simulink model "NDM200"  (Simulink 7.6)
settings: Solver=ode45  StartTime=0.0  StopTime=SimulTime  RelTol=1e-3
values from neighbouring files (symbols this model uses):
  T_amb = 296    [Parameters.m]
undefined symbols (not defined in the file or in its folder): Job
libraries: simulink x1, WZM_QSS_Lib x1
settings Model: Creator=simon  LastModifiedBy=conid
settings DebuggingCC: AlgebraicLoopMsg=none  SolverPrmCheckMsg=none

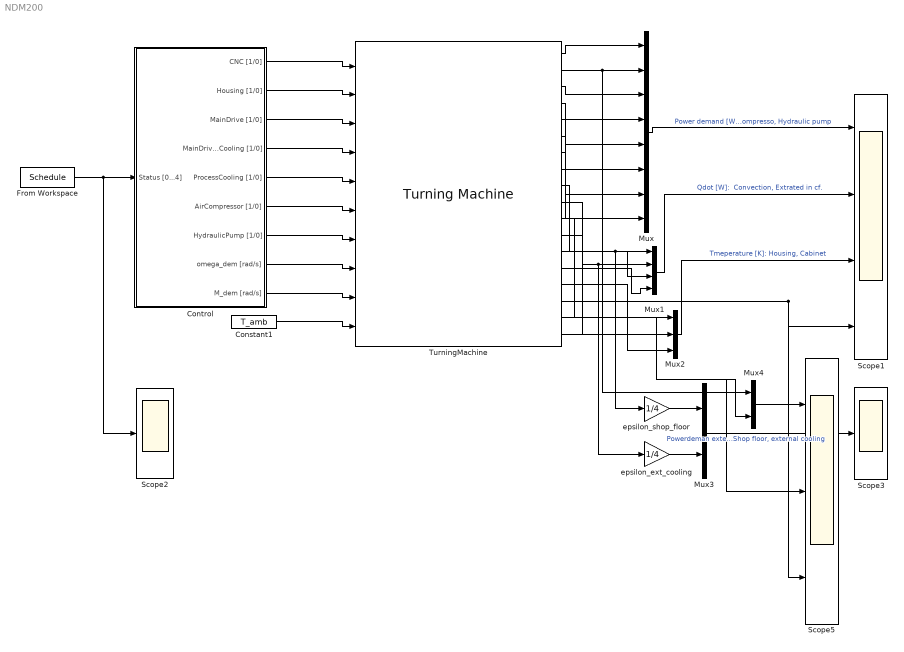
== system NDM200 ==
  Constant1 : Constant  Value=T_amb
  Control : Subsystem  mask{CNC=[0 1 1 1 1], Housing=[0 1 1 1 1], MainDrive=[0 0 0 0 1], MainDriveCooling=[0 0 1 1 1], ProcessCooling=[0 0 0 0 1], AirCompressor=[0 0 1 1 1], HydraulicPump=[0 0 1 1 1], Job=Job}
      mask prompts: CNC "Cabinet"; MainDrive "Main drive"; MainDriveCooling "Main drive cooling"; ProcessCooling "Process cooling"; Job "Job struct"
      mask help:
      | Controls the components of the machine:
      |
      | Status:
      |     0. Off
      |     1. Standby
      |     2. Warmup
      |     3. Setting
      |     4. Machining
      |
      | If the status is machining, the job defined as
      |     - Job.time
      |     - Job.omega_dem
      |     - Job.M_dem
      | will be runned, and repeated.
      mask TabNameString: Status,Status,Status,Status,Status,Status,Status,Job
  From Workspace : FromWorkspace  VariableName=Schedule  SampleTime=0  Interpolate=off  OutputAfterFinalValue=Holding final value
  Mux : Mux  Inputs=8
  Mux1 : Mux
  Mux2 : Mux  Inputs=3
  Mux3 : Mux  Inputs=2
  Mux4 : Mux  Inputs=2
  Scope1 : Scope  NumInputPorts=4
      settings: TickLabels=on  TimeRange=1000  YMin=0~-3e+008~215~-3.25e+010  YMax=200000~1.1e+009~295~2.5e+009  SaveName=Scp_Main
  Scope2 : Scope
      settings: TickLabels=on  TimeRange=350  YMin=0.95  YMax=1.05  SaveName=Scp_Schedule
  Scope3 : Scope
      settings: TickLabels=on  TimeRange=350  YMin=-2.5e+13  YMax=1.25e+13  SaveName=Scp_PwrExt
  Scope5 : Scope  NumInputPorts=3
      settings: TickLabels=on  TimeRange=2000  YMin=0~0~296  YMax=12486.03351955308~5000~306  SaveName=Scp_Main1
  TurningMachine : WZM_QSS_Lib/Assembly/Turning Machine  SystemSampleTime=-1  MainDrive=MainDrive  MainDriveCoolingEx=MainDriveCoolingEx  CNC=CNC  Process=Process  ProcessCooling=ProcessCooling  Housing=Housing  AirCompressor=AirCompressor  HydraulicPump=HydraulicPump  LocMainDrive=machine housing  LocProcessCooling=shop floor  LocProcess=process housing  LocMachine=shop floor  LocMachineExtr=shop floor  LocCNC=shop floor  LocCNCExtr=shop floor  LocAirCompressor=shop floor  LocHydraulicPump=shop floor
      link override MainDrive/MainDrive_simple/Lookup Table (n-D): InterpMethod=Cubic spline
  epsilon_ext_cooling : Gain  Gain=1/4
  epsilon_shop_floor : Gain  Gain=1/4
  wires:
  TurningMachine/1 -> Mux/1
  TurningMachine/2 -> Mux/2, Mux4/1
  TurningMachine/3 -> Mux/3
  TurningMachine/4 -> Mux/4
  TurningMachine/5 -> Mux/5
  TurningMachine/6 -> Mux/6
  Mux/1 -> Scope1/1  "Power demand [W]: Total,  CNC, Main Drive Cooling,  Housing, Process cooling, Cabinet cooling, Air compresso, Hydraulic pump"
  Mux1/1 -> Scope1/2  "Qdot [W]:  Convection, Extrated in cf."
  Mux2/1 -> Scope1/3  "Tmeperature [K]: Housing, Cabinet"
  TurningMachine/7 -> Mux/7
  TurningMachine/8 -> Mux/8
  TurningMachine/9 -> Mux1/1, epsilon_shop_floor/1
  TurningMachine/10 -> epsilon_ext_cooling/1, Mux1/2
  TurningMachine/11 -> Mux2/1
  TurningMachine/12 -> Mux2/2
  Control/1(CNC [1/0]) -> TurningMachine/1
  Control/2(Housing [1/0]) -> TurningMachine/2
  Control/3(MainDrive [1/0]) -> TurningMachine/3
  Control/4(MainDriveCooling [1/0]) -> TurningMachine/4
  Control/5(ProcessCooling [1/0]) -> TurningMachine/5
  Control/6(AirCompressor [1/0]) -> TurningMachine/6
  Control/7(HydraulicPump [1/0]) -> TurningMachine/7
  Control/8(omega_dem [rad/s]) -> TurningMachine/8
  Control/9(M_dem [rad/s]) -> TurningMachine/9
  Constant1/1 -> TurningMachine/10
  From Workspace/1 -> Control/1(Status [0...4]), Scope2/1
  epsilon_shop_floor/1 -> Mux3/1
  epsilon_ext_cooling/1 -> Mux3/2
  Mux3/1 -> Scope3/1  "Powerdeman external components [W]:  Shop floor, external cooling"
  TurningMachine/13 -> Mux1/3
  TurningMachine/14 -> Mux1/4
  TurningMachine/15 -> Mux2/3
  Mux4/1 -> Scope5/1
  TurningMachine/18 -> Mux4/2
  TurningMachine/17 -> Scope5/2
  TurningMachine/16 -> Scope5/3, Scope1/4

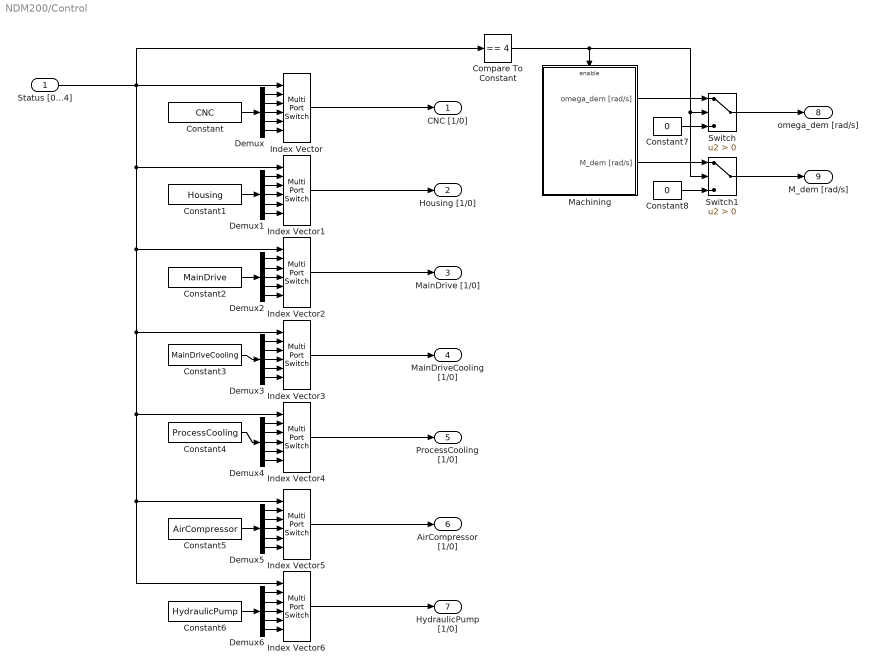
== system NDM200/Control ==
  Status [0...4] : Inport
  Compare To Constant : simulink/Logic and Bit Operations/Compare To Constant  SystemSampleTime=-1  relop===  const=4  LogicOutDataTypeMode=uint8
  Constant : Constant  Value=CNC
  Constant1 : Constant  Value=Housing
  Constant2 : Constant  Value=MainDrive
  Constant3 : Constant  Value=MainDriveCooling
  Constant4 : Constant  Value=ProcessCooling
  Constant5 : Constant  Value=AirCompressor
  Constant6 : Constant  Value=HydraulicPump
  Constant7 : Constant  Value=0
  Constant8 : Constant  Value=0
  Demux{,1..6} (7 alike) : Demux  Outputs=5
  Index Vector{,1..6} (7 alike) : MultiPortSwitch  DataPortOrder=Zero-based contiguous  Inputs=5  zeroidx=on
  Machining : Subsystem  TreatAsAtomicUnit=on
  Switch : Switch  Criteria=u2 > Threshold
  Switch1 : Switch  Criteria=u2 > Threshold
  CNC [1/0] : Outport
  Housing [1/0] : Outport  Port=2
  MainDrive [1/0] : Outport  Port=3
  MainDriveCooling [1/0] : Outport  Port=4
  ProcessCooling [1/0] : Outport  Port=5
  AirCompressor [1/0] : Outport  Port=6
  HydraulicPump [1/0] : Outport  Port=7
  omega_dem [rad/s] : Outport  Port=8
  M_dem [rad/s] : Outport  Port=9
  wires:
  Status [0...4]/1 -> Index Vector/1, Index Vector1/1, Index Vector2/1, Index Vector3/1, Index Vector4/1, Index Vector5/1, Index Vector6/1, Compare To Constant/1
  Demux/1 -> Index Vector/2
  Demux/2 -> Index Vector/3
  Demux/3 -> Index Vector/4
  Demux/4 -> Index Vector/5
  Demux/5 -> Index Vector/6
  Constant/1 -> Demux/1
  Index Vector/1 -> CNC [1/0]/1
  Demux1/1 -> Index Vector1/2
  Demux1/2 -> Index Vector1/3
  Demux1/3 -> Index Vector1/4
  Demux1/4 -> Index Vector1/5
  Demux1/5 -> Index Vector1/6
  Constant1/1 -> Demux1/1
  Demux2/1 -> Index Vector2/2
  Demux2/2 -> Index Vector2/3
  Demux2/3 -> Index Vector2/4
  Demux2/4 -> Index Vector2/5
  Demux2/5 -> Index Vector2/6
  Constant2/1 -> Demux2/1
  Demux3/1 -> Index Vector3/2
  Demux3/2 -> Index Vector3/3
  Demux3/3 -> Index Vector3/4
  Demux3/4 -> Index Vector3/5
  Demux3/5 -> Index Vector3/6
  Constant3/1 -> Demux3/1
  Index Vector1/1 -> Housing [1/0]/1
  Index Vector2/1 -> MainDrive [1/0]/1
  Index Vector3/1 -> MainDriveCooling [1/0]/1
  Demux4/1 -> Index Vector4/2
  Demux4/2 -> Index Vector4/3
  Demux4/3 -> Index Vector4/4
  Demux4/4 -> Index Vector4/5
  Demux4/5 -> Index Vector4/6
  Constant4/1 -> Demux4/1
  Demux5/1 -> Index Vector5/2
  Demux5/2 -> Index Vector5/3
  Demux5/3 -> Index Vector5/4
  Demux5/4 -> Index Vector5/5
  Demux5/5 -> Index Vector5/6
  Constant5/1 -> Demux5/1
  Demux6/1 -> Index Vector6/2
  Demux6/2 -> Index Vector6/3
  Demux6/3 -> Index Vector6/4
  Demux6/4 -> Index Vector6/5
  Demux6/5 -> Index Vector6/6
  Constant6/1 -> Demux6/1
  Index Vector4/1 -> ProcessCooling [1/0]/1
  Index Vector5/1 -> AirCompressor [1/0]/1
  Index Vector6/1 -> HydraulicPump [1/0]/1
  Compare To Constant/1 -> Machining/Enable, Switch/2, Switch1/2
  Machining/1(omega_dem [rad/s]) -> Switch/1
  Machining/2(M_dem [rad/s]) -> Switch1/1
  Switch/1 -> omega_dem [rad/s]/1
  Switch1/1 -> M_dem [rad/s]/1
  Constant7/1 -> Switch/3
  Constant8/1 -> Switch1/3

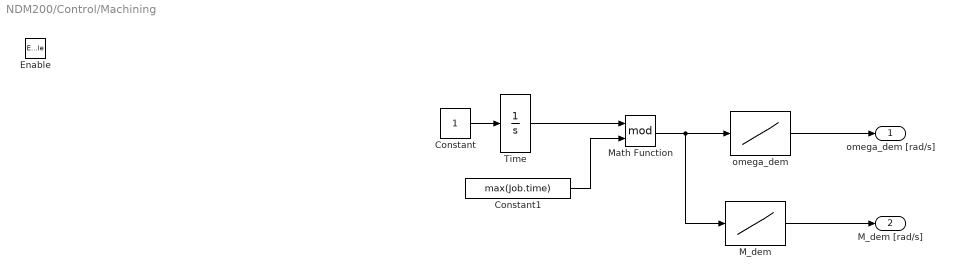
== system NDM200/Control/Machining ==
  Enable : EnablePort  StatesWhenEnabling=reset
  Constant : Constant
  Constant1 : Constant  Value=max(Job.time)
  M_dem : Lookup_n-D  NumberOfTableDimensions=1  BreakpointsForDimension1=Job.time  Table=Job.M_dem  InterpMethod=None - Flat  ExtrapMethod=Cubic spline  RndMeth=Simplest  InputSameDT=on
  Math Function : Math  Operator=mod  SaturateOnIntegerOverflow=on
  Time : Integrator
  omega_dem : Lookup_n-D  NumberOfTableDimensions=1  BreakpointsForDimension1=Job.time  Table=Job.omega_dem  InterpMethod=None - Flat  ExtrapMethod=Cubic spline  RndMeth=Simplest  InputSameDT=on
  omega_dem [rad/s] : Outport
  M_dem [rad/s] : Outport  Port=2
  wires:
  Constant/1 -> Time/1
  omega_dem/1 -> omega_dem [rad/s]/1
  M_dem/1 -> M_dem [rad/s]/1
  Math Function/1 -> omega_dem/1, M_dem/1
  Time/1 -> Math Function/1
  Constant1/1 -> Math Function/2
